simulink model "adaptive_observer_for_sin_signal_original"  (R2021b)
settings: Solver=ode4  StartTime=0.0  StopTime=simulationTime  FixedStep=0.0001  RelTol=1e-3
model workspace: external: MATLAB File D:\practice\sci\variables2n1.m (data not in the file)
values from neighbouring files (symbols this model uses):
  A = zeros(2*dimension+1 , 2*dimension+1)    [LCAD.m]
  alpha = [1,3]    [variables2n1.m]
  amp = [1;1]    [variables2n1.m]
  amp_M = [1;1]    [variables2n1.m]
  amp_M1 = 0.2    [variables2n1.m]
  bias = [0;0]    [variables2n1.m]
  bias_M = [0;0]    [variables2n1.m]
  bias_M1 = 0    [variables2n1.m]
  bigGammaZ0 = zeros(2*dimension+1, dimension)    [variables2n1.m]
  C = zeros(1, 2*dimension+1)    [LCAD.m]
  delta = C*A    [LCAD.m]    (also in stats.m = 0.05)
  dimension = 2    [variables2n1.m]
  freq = [2;3]    [variables2n1.m]
  freq_M = [1.8;3.2]    [variables2n1.m]
  freq_M1 = 20    [variables2n1.m]
  freqSwitcher = [80,150]    [variables2n1.m]
  gamma_my = 0.01    [starter3.m]
  h_my = 0.3    [starter3.m]
  initialTheta = [initialOmega(1)^2-alpha(1);     initialOmega(2)^2-alpha(2)]    [variables2n1.m]
  initialZ = [sin(phase(1)); r^2*cos(phase(1))/initialOmega(1);     sin(phase(2)); r^2*cos(phase(2))/initialOmega(2); sum(bias)]    [variables2n1.m]
  k_my = 100    [starter3.m]
  L = real((place(A',C',eigenvalues))')    [LCAD.m]
  mu = 25    [graphs.m]    (also in plot_pres4.m = 2.5; variables2n1.m = 2.5)
  noiseOrSin = 0    [variables2n1.m]
  noiseOrSwitch = 0    [variables2n1.m]
  omega1 = ones(1, length(time))*2    [graphs.m]    (also in starter3.m = 2)
  omega2 = ones(1, length(time))*3    [graphs.m]    (also in starter3.m = 3)
  omega_max = 10    [starter3.m]
  omega_min = 1    [starter3.m]
  omegaLimiter = sqrt(dimension)*maxOmega    [variables2n1.m]
  phase = [0;0]    [variables2n1.m]
  phase_M = [0;0]    [variables2n1.m]
  phase_M1 = 0    [variables2n1.m]
  r = 1.2    [variables2n1.m]
  sample_M1 = 10    [variables2n1.m]
  tau_my = 0.3    [starter3.m]
  theta0_my = [-2; 1]    [starter3.m]
  theta_real = [-c1-c2; c1*c2]    [starter3.m]
  turn_mods_on = 1    [variables2n1.m]
  zMax = 5    [variables2n1.m]
undefined symbols (not defined in the file or in its folder): G, isComplex, L1
libraries: simulink x1
(part 2 of 3)

== system adaptive_observer_for_sin_signal_original/Proposed Estimator/Subsystem ==
  Ω : Inport
  Constant1 : Constant  Value=r^2
  Divide : Product  Inputs=*/
  Gain1 : Gain  Gain=r^2
  Transpose{,1..3} (4 alike) : Math  Operator=transpose  SaturateOnIntegerOverflow=on
  Λ : Constant  Value=alpha
  Ω-Λ : Sum  Inputs=+-
  Ф : Outport
  wires:
  Divide/1 -> Ω-Λ/1
  Ω-Λ/1 -> Transpose1/1
  Ω/1 -> Divide/1
  Constant1/1 -> Divide/2
  Gain1/1 -> Transpose2/1
  Λ/1 -> Transpose/1
  Transpose/1 -> Gain1/1
  Transpose2/1 -> Ω-Λ/2
  Transpose1/1 -> Transpose3/1
  Transpose3/1 -> Ф/1

== system adaptive_observer_for_sin_signal_original/Proposed Estimator/Subsystem1 ==
  u : Inport
  Complex to Real-Imag : ComplexToRealImag
  MATLAB Function : MATLAB Function  TreatAsAtomicUnit=on
  Real-Imag to Complex : RealImagToComplex
  Switcher : Switch  Criteria=u2 ~= 0  Threshold=freqSwitcher(1)
  isComplex : Constant  Value=isComplex
  "∫Z " : Integrator  Priority=1  InitialCondition=real(initialZ)
  ∫Z 1 : Integrator  Priority=1  InitialCondition=imag(initialZ)
  Out1 : Outport
  wires:
  isComplex/1 -> Switcher/2
  u/1 -> MATLAB Function/1(zPrime), Complex to Real-Imag/1
  "∫Z "/1 -> Real-Imag to Complex/1, Switcher/1
  Switcher/1 -> Out1/1
  Complex to Real-Imag/1 -> "∫Z "/1
  Complex to Real-Imag/2 -> ∫Z 1/1
  ∫Z 1/1 -> Real-Imag to Complex/2
  Real-Imag to Complex/1 -> Switcher/3

== system adaptive_observer_for_sin_signal_original/Proposed Estimator/z' ==
  y : Inport
  Г(z) : Inport  Port=2
  Ф : Inport  Port=3
  z : Inport  Port=4
  Minus : Sum  Inputs=+-
  Product : Product  Multiplication=Matrix(*)
  S(z) : Subsystem
  Subsystem : Subsystem
  z' : Outport
  wires:
  z/1 -> Subsystem/4(z), S(z)/2(z)
  Minus/1 -> z'/1
  S(z)/1(S) -> Product/1
  Product/1 -> Minus/2
  Subsystem/1(zPreDot) -> Minus/1, Product/2, S(z)/1(zPreDot)
  Г(z)/1 -> Subsystem/1(bigGamma)
  Ф/1 -> Subsystem/2(PHI)
  y/1 -> Subsystem/3(y)

== system adaptive_observer_for_sin_signal_original/Proposed Estimator1/Frequencies estimator ==
  Ф : Inport
  ż : Inport  Port=2
  Ω in : Inport  Port=3
  z : Inport  Port=4
  y : Inport  Port=5
  Fc : Subsystem  Priority=8  TreatAsAtomicUnit=on
      settings: PortSchema="{\"entries\":[{\"content\":{\"sides\":[{\"content\":{\"connectorIds\":[\"In1\",\"In2\",\"In3\"]},\"type\":\"ConnectorPlacement.EquallySpacedRectSide\",\"uuid\":\"ef8cffdc-1e6f-42c0-8cb3-bf318ca182f8\"},{\"content\":{\"connectorIds\":[\"Out1\"],\"side\":\"RIGHT\"},\"type\":\"ConnectorPlacement.EquallySpacedRectSide\",\"uuid\":\"a9c7e5b7-281a-47aa-808a-eb2877f3eee0\"},{\"content\":{\"connectorIds\":[\"In4\"],\"side\":\"TOP\"},\"type\":\"ConnectorPlacement.EquallySpacedRectSide\",\"uuid\":\"7bb4f6b5-7deb-4e08-9b2d-b96cfbb2c85e\"},{\"content\":{\"connectorIds\":[],\"side\":\"BOTTOM\"},\"type\":\"ConnectorPlacement.EquallySpacedRectSide\",\"uuid\":\"d628d464-6f95-4c60-8de5-a9188665a8a2\"}]},\"type\":\"ConnectorPlacement.EquallySpacedConnector\",\"uuid\":\"64fccc24-315d-40ff-920f-bd434d551c1a\"}],\"packageUris\":[\"http://schema.mathworks.com/mf0/Connector/R2020b\"],\"version\":\"1.0\"}"
  Fu : Subsystem  Priority=9  TreatAsAtomicUnit=on
      settings: PortSchema="{\"entries\":[{\"content\":{\"sides\":[{\"content\":{\"connectorIds\":[\"In1\",\"In2\"]},\"type\":\"ConnectorPlacement.EquallySpacedRectSide\",\"uuid\":\"56415c13-d553-4f88-94d3-75bcdc800e4b\"},{\"content\":{\"connectorIds\":[\"Out1\"],\"side\":\"RIGHT\"},\"type\":\"ConnectorPlacement.EquallySpacedRectSide\",\"uuid\":\"a1bdd2d2-4e49-40cb-b0b7-1df5316e4510\"},{\"content\":{\"connectorIds\":[\"In3\"],\"side\":\"TOP\"},\"type\":\"ConnectorPlacement.EquallySpacedRectSide\",\"uuid\":\"59b6ba3d-4a55-43e8-9b14-0d873cc3c9ca\"},{\"content\":{\"connectorIds\":[\"In4\",\"In5\"],\"side\":\"BOTTOM\"},\"type\":\"ConnectorPlacement.EquallySpacedRectSide\",\"uuid\":\"cb3db39e-f643-4fe7-a27f-76e86359c78d\"}]},\"type\":\"ConnectorPlacement.EquallySpacedConnector\",\"uuid\":\"fdf2e112-ecff-41aa-a5cb-d527a9dd51a8\"}],\"packageUris\":[\"http://schema.mathworks.com/mf0/Connector/R2020b\"],\"version\":\"1.0\"}"
  Ω : Subsystem  Priority=5  TreatAsAtomicUnit=on
      settings: PortSchema="{\"entries\":[{\"content\":{\"sides\":[{\"content\":{\"connectorIds\":[\"In1\",\"In2\"]},\"type\":\"ConnectorPlacement.EquallySpacedRectSide\",\"uuid\":\"0172ca52-64e8-432c-895c-e5829558e278\"},{\"content\":{\"connectorIds\":[\"Out1\"],\"side\":\"RIGHT\"},\"type\":\"ConnectorPlacement.EquallySpacedRectSide\",\"uuid\":\"c83f4e01-5d94-498a-a9de-b4a302d500ab\"},{\"content\":{\"connectorIds\":[\"In3\"],\"side\":\"TOP\"},\"type\":\"ConnectorPlacement.EquallySpacedRectSide\",\"uuid\":\"3a6496e3-470c-4361-9f8f-cd28e1556398\"}]},\"type\":\"ConnectorPlacement.EquallySpacedConnector\",\"uuid\":\"b738ec8a-20ee-4a0a-8362-4988f331d970\"}],\"packageUris\":[\"http://schema.mathworks.com/mf0/Connector/R2020b\"],\"version\":\"1.0\"}"
  θ' : Subsystem  Priority=10  TreatAsAtomicUnit=on
      settings: PortSchema="{\"entries\":[{\"content\":{\"sides\":[{\"content\":{\"connectorIds\":[\"In1\"]},\"type\":\"ConnectorPlacement.EquallySpacedRectSide\",\"uuid\":\"9184f415-d771-478b-8114-38f854f6aad6\"},{\"content\":{\"connectorIds\":[\"Out1\"],\"side\":\"RIGHT\"},\"type\":\"ConnectorPlacement.EquallySpacedRectSide\",\"uuid\":\"399c2935-e635-4d1c-9ba7-451eea57bae3\"},{\"content\":{\"connectorIds\":[\"In2\"],\"side\":\"TOP\"},\"type\":\"ConnectorPlacement.EquallySpacedRectSide\",\"uuid\":\"bdc6ec05-8dca-4996-ba70-702aa29fd179\"}]},\"type\":\"ConnectorPlacement.EquallySpacedConnector\",\"uuid\":\"fa68c3f3-8285-4ee8-b99d-908dba81143c\"}],\"packageUris\":[\"http://schema.mathworks.com/mf0/Connector/R2020b\"],\"version\":\"1.0\"}"
  г(z) : Selector  InputPortWidth=2*dimension+1  IndexOptions=Index vector (dialog)  Indices=2:2:2*dimension  OutputSizes=1
  "∫θ " : Integrator  Priority=3  InitialCondition=initialTheta
  Ω out : Outport
  wires:
  Ф/1 -> Fu/1(Ф), Fc/3(Ф)
  y/1 -> Ω/2(y), Fu/5(y)
  z/1 -> г(z)/1, Fu/2(z), Fc/1(z)
  г(z)/1 -> Fc/4(Г(z)), Ω/3(г(z)), Fu/4(г(z))
  Ω in/1 -> Fc/2(Ω)
  ż/1 -> Fu/3(ż)
  "∫θ "/1 -> Ω/1(θ)
  Ω/1(Ω) -> Ω out/1
  Fc/1(Fc) -> θ'/2(Fc)
  Fu/1(Fu) -> θ'/1(Fu)
  θ'/1(θ') -> "∫θ "/1

== system adaptive_observer_for_sin_signal_original/Proposed Estimator1/Subsystem ==
  Ω : Inport
  Constant1 : Constant  Value=r^2
  Divide : Product  Inputs=*/
  Gain1 : Gain  Gain=r^2
  Transpose{,1..3} (4 alike) : Math  Operator=transpose  SaturateOnIntegerOverflow=on
  Λ : Constant  Value=alpha
  Ω-Λ : Sum  Inputs=+-
  Ф : Outport
  wires:
  Divide/1 -> Ω-Λ/1
  Ω-Λ/1 -> Transpose1/1
  Ω/1 -> Divide/1
  Constant1/1 -> Divide/2
  Gain1/1 -> Transpose2/1
  Λ/1 -> Transpose/1
  Transpose/1 -> Gain1/1
  Transpose2/1 -> Ω-Λ/2
  Transpose1/1 -> Transpose3/1
  Transpose3/1 -> Ф/1

== system adaptive_observer_for_sin_signal_original/Proposed Estimator1/Subsystem1 ==
  u : Inport
  Complex to Real-Imag : ComplexToRealImag
  MATLAB Function : MATLAB Function  TreatAsAtomicUnit=on
  Real-Imag to Complex : RealImagToComplex
  Switcher : Switch  Criteria=u2 ~= 0  Threshold=freqSwitcher(1)
  isComplex : Constant  Value=isComplex
  "∫Z " : Integrator  Priority=1  InitialCondition=real(initialZ)
  ∫Z 1 : Integrator  Priority=1  InitialCondition=imag(initialZ)
  Out1 : Outport
  wires:
  isComplex/1 -> Switcher/2
  u/1 -> MATLAB Function/1(zPrime), Complex to Real-Imag/1
  "∫Z "/1 -> Real-Imag to Complex/1, Switcher/1
  Switcher/1 -> Out1/1
  Complex to Real-Imag/1 -> "∫Z "/1
  Complex to Real-Imag/2 -> ∫Z 1/1
  ∫Z 1/1 -> Real-Imag to Complex/2
  Real-Imag to Complex/1 -> Switcher/3

== system adaptive_observer_for_sin_signal_original/Proposed Estimator1/z' ==
  y : Inport
  Г(z) : Inport  Port=2
  Ф : Inport  Port=3
  z : Inport  Port=4
  Minus : Sum  Inputs=+-
  Product : Product  Multiplication=Matrix(*)
  S(z) : Subsystem
  Subsystem : Subsystem
  z' : Outport
  wires:
  z/1 -> Subsystem/4(z), S(z)/2(z)
  Minus/1 -> z'/1
  S(z)/1(S) -> Product/1
  Product/1 -> Minus/2
  Subsystem/1(zPreDot) -> Minus/1, Product/2, S(z)/1(zPreDot)
  Г(z)/1 -> Subsystem/1(bigGamma)
  Ф/1 -> Subsystem/2(PHI)
  y/1 -> Subsystem/3(y)

== system adaptive_observer_for_sin_signal_original/Estimator mu=10/Frequencies estimator/Fc ==
  note: Определение максимального S
  note: Переключатель ограничителя Fc
  z : Inport
  Ω : Inport  Port=2
  Ф : Inport  Port=3
  Г(z) : Inport  Port=4
  Clock : Clock
  Constant : Constant  Value=mu(4)
  Scope2 : Scope
  Unary Minus : UnaryMinus
  max S1 : MATLAB Function  TreatAsAtomicUnit=on
  product : Product  Inputs=3
  ||Ω|| : MATLAB Function  TreatAsAtomicUnit=on
  "||Ω|| >= Ω cap ? " : RelationalOperator  OutDataTypeStr=boolean  RndMeth=Simplest
  Ψ : MATLAB Function  TreatAsAtomicUnit=on
  Ω * √n : Constant  Value=omegaLimiter
  Ω / Ω cap : Product  Inputs=*/
  Fc : Outport
  wires:
  Ф/1 -> max S1/3(PHI)
  Ω/1 -> max S1/1(bigOmega), Ω / Ω cap/1, ||Ω||/1(bigOmega)
  max S1/1(maxS) -> product/3, Scope2/1
  Г(z)/1 -> max S1/4(gammaZ)
  z/1 -> max S1/2(z)
  ||Ω||/1(normOmega) -> "||Ω|| >= Ω cap ? "/1
  Ω * √n/1 -> Ω / Ω cap/2, "||Ω|| >= Ω cap ? "/2
  "||Ω|| >= Ω cap ? "/1 -> Ψ/1(isGreater)
  Ψ/1(Psi) -> product/1
  Ω / Ω cap/1 -> product/2
  product/1 -> Unary Minus/1
  Unary Minus/1 -> Fc/1
  Clock/1 -> max S1/5(t)
  Constant/1 -> max S1/6(mu)

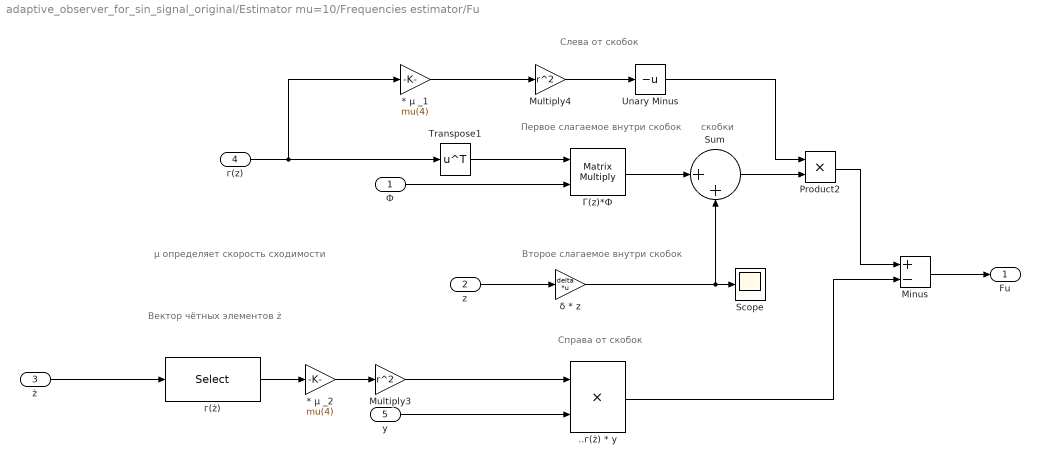
== system adaptive_observer_for_sin_signal_original/Estimator mu=10/Frequencies estimator/Fu ==
  note: Вектор чётных элементов ż
  note: μ определяет скорость сходимости
  note: скобки
  note: Первое слагаемое внутри скобок
  note: Второе слагаемое внутри скобок
  note: Слева от скобок
  note: Справа от скобок
  Ф : Inport
  z : Inport  Port=2
  ż : Inport  Port=3
  г(z) : Inport  Port=4
  y : Inport  Port=5
  * μ _1 : Gain  Gain=mu(4)
  * μ _2 : Gain  Gain=mu(4)
  ..г(ż) * y : Product
  Minus : Sum  Inputs=+-
  Multiply3 : Gain  Gain=r^2
  Multiply4 : Gain  Gain=r^2
  Product2 : Product
  Scope : Scope
  Sum : Sum  Inputs=|++
  Transpose1 : Math  Operator=transpose  SaturateOnIntegerOverflow=on
  Unary Minus : UnaryMinus
  δ * z : Gain  Gain=delta  Multiplication=Matrix(K*u)
  Г(z)*Ф : Product  Multiplication=Matrix(*)
  г(ż) : Selector  InputPortWidth=2*dimension+1  IndexOptions=Index vector (dialog)  Indices=2:2:2*dimension  OutputSizes=1
  Fu : Outport
  wires:
  ż/1 -> г(ż)/1
  г(z)/1 -> * μ _1/1, Transpose1/1
  * μ _2/1 -> Multiply3/1
  г(ż)/1 -> * μ _2/1
  Multiply3/1 -> ..г(ż) * y/1
  y/1 -> ..г(ż) * y/2
  Transpose1/1 -> Г(z)*Ф/1
  * μ _1/1 -> Multiply4/1
  Multiply4/1 -> Unary Minus/1
  z/1 -> δ * z/1
  Г(z)*Ф/1 -> Sum/1
  δ * z/1 -> Scope/1, Sum/2
  Unary Minus/1 -> Product2/1
  Sum/1 -> Product2/2
  Product2/1 -> Minus/1
  ..г(ż) * y/1 -> Minus/2
  Minus/1 -> Fu/1
  Ф/1 -> Г(z)*Ф/2

== system adaptive_observer_for_sin_signal_original/Estimator mu=10/Frequencies estimator/Ω ==
  note: Оценка частот в момент времени t
  θ : Inport
  y : Inport  Port=2
  г(z) : Inport  Port=3
  ..г(z)*y : Product
  Gain : Gain  Gain=r^2
  Sum : Sum  Inputs=|++
  μ : Gain  Gain=mu(4)
  Ω : Outport
  wires:
  г(z)/1 -> Gain/1
  Gain/1 -> μ/1
  μ/1 -> ..г(z)*y/1
  y/1 -> ..г(z)*y/2
  ..г(z)*y/1 -> Sum/1
  θ/1 -> Sum/2
  Sum/1 -> Ω/1

== system adaptive_observer_for_sin_signal_original/Estimator mu=10/Frequencies estimator/θ' ==
  note: Образует основу θ'
  note: Удерживает Ω в области определения
  Fu : Inport
  Fc : Inport  Port=2
  Sum : Sum  Inputs=|++
  θ' : Outport
  wires:
  Fu/1 -> Sum/2
  Sum/1 -> θ'/1
  Fc/1 -> Sum/1

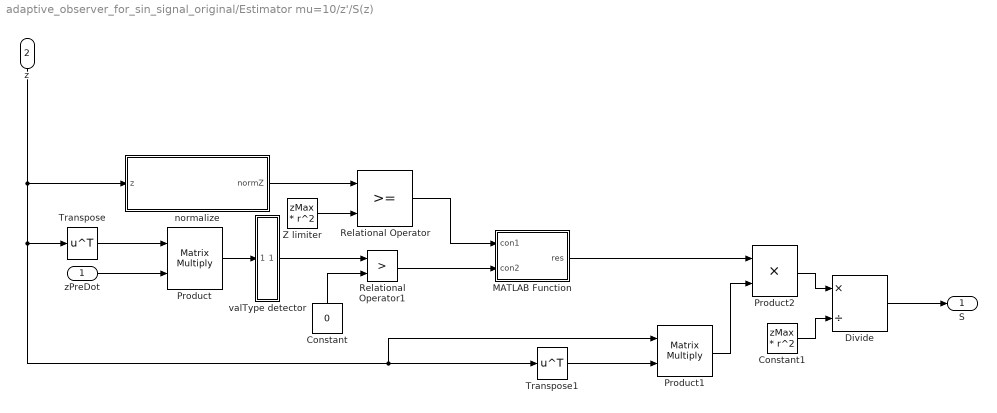
== system adaptive_observer_for_sin_signal_original/Estimator mu=10/z'/S(z) ==
  zPreDot : Inport
  z : Inport  Port=2
  Constant : Constant  Value=0
  Constant1 : Constant  Value=zMax * r^2
  Divide : Product  Inputs=*/
  MATLAB Function : MATLAB Function  TreatAsAtomicUnit=on
  Product : Product  Multiplication=Matrix(*)
  Product1 : Product  Multiplication=Matrix(*)
  Product2 : Product
  Relational Operator : RelationalOperator  OutDataTypeStr=boolean  RndMeth=Simplest
  Relational Operator1 : RelationalOperator  Operator=>  OutDataTypeStr=boolean  RndMeth=Simplest
  Transpose : Math  Operator=transpose  SaturateOnIntegerOverflow=on
  Transpose1 : Math  Operator=transpose  SaturateOnIntegerOverflow=on
  Z limiter : Constant  Value=zMax * r^2
  normalize : MATLAB Function  TreatAsAtomicUnit=on
  valType detector : MATLAB Function  TreatAsAtomicUnit=on
  S : Outport
  wires:
  Z limiter/1 -> Relational Operator/2
  normalize/1(normZ) -> Relational Operator/1
  Relational Operator/1 -> MATLAB Function/1(con1)
  z/1 -> Product1/1, Transpose1/1, Transpose/1, normalize/1(z)
  Transpose/1 -> Product/1
  zPreDot/1 -> Product/2
  Product/1 -> valType detector/1(multiplied)
  Constant/1 -> Relational Operator1/2
  Relational Operator1/1 -> MATLAB Function/2(con2)
  MATLAB Function/1(res) -> Product2/1
  Transpose1/1 -> Product1/2
  Product1/1 -> Product2/2
  Product2/1 -> Divide/1
  Constant1/1 -> Divide/2
  Divide/1 -> S/1
  valType detector/1(filtered) -> Relational Operator1/1

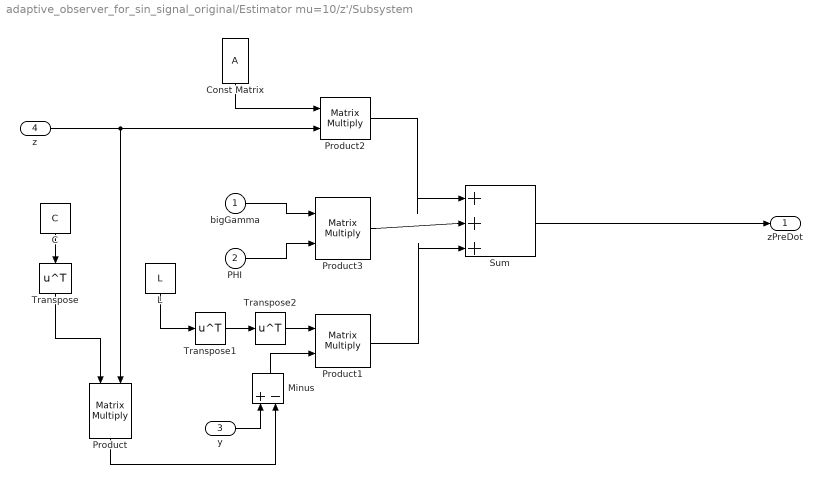
== system adaptive_observer_for_sin_signal_original/Estimator mu=10/z'/Subsystem ==
  bigGamma : Inport
  PHI : Inport  Port=2
  y : Inport  Port=3
  z : Inport  Port=4
  C : Constant  Value=C
  Const Matrix : Constant  Value=A
  L : Constant  Value=L
  Minus : Sum  Inputs=+-
  Product{,1..3} (4 alike) : Product  Multiplication=Matrix(*)
  Sum : Sum  Inputs=|+++
  Transpose : Math  Operator=transpose  SaturateOnIntegerOverflow=on
  Transpose1 : Math  Operator=transpose  SaturateOnIntegerOverflow=on
  Transpose2 : Math  Operator=transpose  SaturateOnIntegerOverflow=on
  zPreDot : Outport
  wires:
  z/1 -> Product2/2, Product/2
  Sum/1 -> zPreDot/1
  C/1 -> Transpose/1
  y/1 -> Minus/1
  Product/1 -> Minus/2
  L/1 -> Transpose1/1
  Minus/1 -> Product1/2
  Const Matrix/1 -> Product2/1
  bigGamma/1 -> Product3/1
  PHI/1 -> Product3/2
  Product2/1 -> Sum/1
  Product3/1 -> Sum/2
  Product1/1 -> Sum/3
  Transpose/1 -> Product/1
  Transpose2/1 -> Product1/1
  Transpose1/1 -> Transpose2/1

== system adaptive_observer_for_sin_signal_original/Estimator mu=2.5/Frequencies estimator/Fc ==
  note: Определение максимального S
  note: Переключатель ограничителя Fc
  z : Inport
  Ω : Inport  Port=2
  Ф : Inport  Port=3
  Г(z) : Inport  Port=4
  Clock : Clock
  Constant : Constant  Value=mu(2)
  Scope2 : Scope
  Unary Minus : UnaryMinus
  max S1 : MATLAB Function  TreatAsAtomicUnit=on
  product : Product  Inputs=3
  ||Ω|| : MATLAB Function  TreatAsAtomicUnit=on
  "||Ω|| >= Ω cap ? " : RelationalOperator  OutDataTypeStr=boolean  RndMeth=Simplest
  Ψ : MATLAB Function  TreatAsAtomicUnit=on
  Ω * √n : Constant  Value=omegaLimiter
  Ω / Ω cap : Product  Inputs=*/
  Fc : Outport
  wires:
  Ф/1 -> max S1/3(PHI)
  Ω/1 -> max S1/1(bigOmega), Ω / Ω cap/1, ||Ω||/1(bigOmega)
  max S1/1(maxS) -> product/3, Scope2/1
  Г(z)/1 -> max S1/4(gammaZ)
  z/1 -> max S1/2(z)
  ||Ω||/1(normOmega) -> "||Ω|| >= Ω cap ? "/1
  Ω * √n/1 -> Ω / Ω cap/2, "||Ω|| >= Ω cap ? "/2
  "||Ω|| >= Ω cap ? "/1 -> Ψ/1(isGreater)
  Ψ/1(Psi) -> product/1
  Ω / Ω cap/1 -> product/2
  product/1 -> Unary Minus/1
  Unary Minus/1 -> Fc/1
  Clock/1 -> max S1/5(t)
  Constant/1 -> max S1/6(mu)

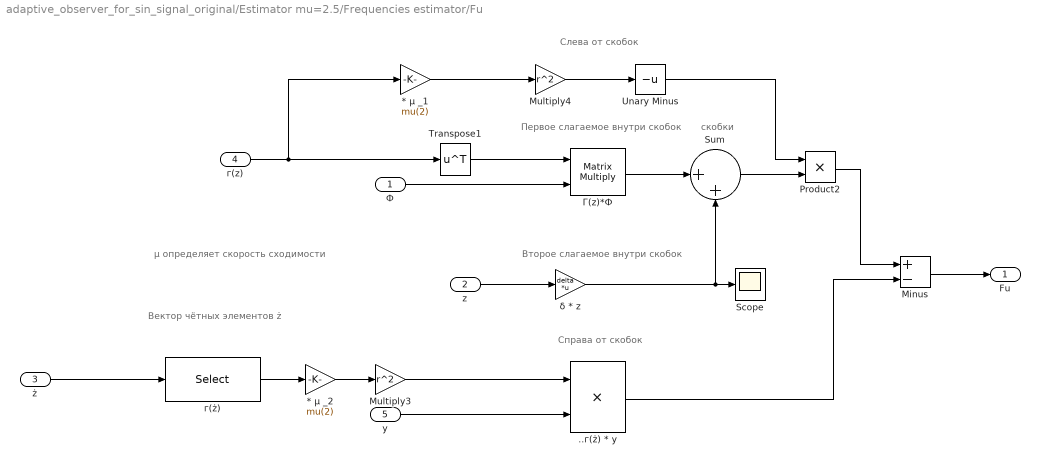
== system adaptive_observer_for_sin_signal_original/Estimator mu=2.5/Frequencies estimator/Fu ==
  note: Вектор чётных элементов ż
  note: μ определяет скорость сходимости
  note: скобки
  note: Первое слагаемое внутри скобок
  note: Второе слагаемое внутри скобок
  note: Слева от скобок
  note: Справа от скобок
  Ф : Inport
  z : Inport  Port=2
  ż : Inport  Port=3
  г(z) : Inport  Port=4
  y : Inport  Port=5
  * μ _1 : Gain  Gain=mu(2)
  * μ _2 : Gain  Gain=mu(2)
  ..г(ż) * y : Product
  Minus : Sum  Inputs=+-
  Multiply3 : Gain  Gain=r^2
  Multiply4 : Gain  Gain=r^2
  Product2 : Product
  Scope : Scope
  Sum : Sum  Inputs=|++
  Transpose1 : Math  Operator=transpose  SaturateOnIntegerOverflow=on
  Unary Minus : UnaryMinus
  δ * z : Gain  Gain=delta  Multiplication=Matrix(K*u)
  Г(z)*Ф : Product  Multiplication=Matrix(*)
  г(ż) : Selector  InputPortWidth=2*dimension+1  IndexOptions=Index vector (dialog)  Indices=2:2:2*dimension  OutputSizes=1
  Fu : Outport
  wires:
  ż/1 -> г(ż)/1
  г(z)/1 -> * μ _1/1, Transpose1/1
  * μ _2/1 -> Multiply3/1
  г(ż)/1 -> * μ _2/1
  Multiply3/1 -> ..г(ż) * y/1
  y/1 -> ..г(ż) * y/2
  Transpose1/1 -> Г(z)*Ф/1
  * μ _1/1 -> Multiply4/1
  Multiply4/1 -> Unary Minus/1
  z/1 -> δ * z/1
  Г(z)*Ф/1 -> Sum/1
  δ * z/1 -> Scope/1, Sum/2
  Unary Minus/1 -> Product2/1
  Sum/1 -> Product2/2
  Product2/1 -> Minus/1
  ..г(ż) * y/1 -> Minus/2
  Minus/1 -> Fu/1
  Ф/1 -> Г(z)*Ф/2

== system adaptive_observer_for_sin_signal_original/Estimator mu=2.5/Frequencies estimator/Ω ==
  note: Оценка частот в момент времени t
  θ : Inport
  y : Inport  Port=2
  г(z) : Inport  Port=3
  ..г(z)*y : Product
  Gain : Gain  Gain=r^2
  Sum : Sum  Inputs=|++
  μ : Gain  Gain=mu(2)
  Ω : Outport
  wires:
  г(z)/1 -> Gain/1
  Gain/1 -> μ/1
  μ/1 -> ..г(z)*y/1
  y/1 -> ..г(z)*y/2
  ..г(z)*y/1 -> Sum/1
  θ/1 -> Sum/2
  Sum/1 -> Ω/1

== system adaptive_observer_for_sin_signal_original/Estimator mu=2.5/Frequencies estimator/θ' ==
  note: Образует основу θ'
  note: Удерживает Ω в области определения
  Fu : Inport
  Fc : Inport  Port=2
  Sum : Sum  Inputs=|++
  θ' : Outport
  wires:
  Fu/1 -> Sum/2
  Sum/1 -> θ'/1
  Fc/1 -> Sum/1

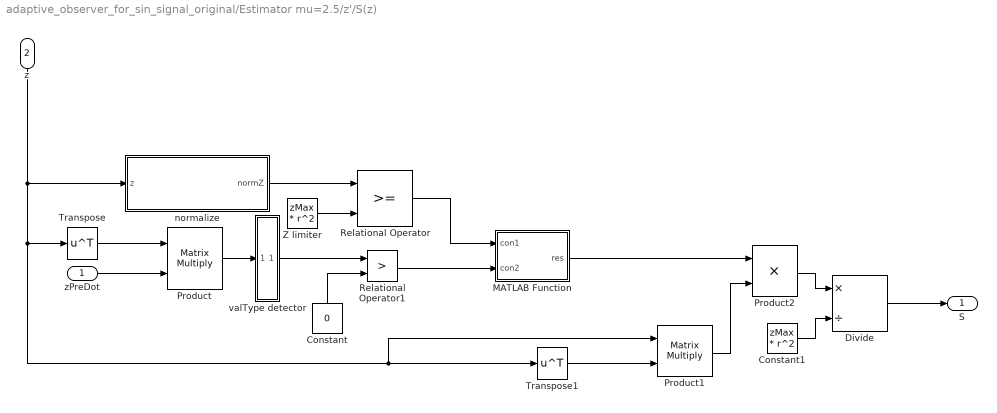
== system adaptive_observer_for_sin_signal_original/Estimator mu=2.5/z'/S(z) ==
  zPreDot : Inport
  z : Inport  Port=2
  Constant : Constant  Value=0
  Constant1 : Constant  Value=zMax * r^2
  Divide : Product  Inputs=*/
  MATLAB Function : MATLAB Function  TreatAsAtomicUnit=on
  Product : Product  Multiplication=Matrix(*)
  Product1 : Product  Multiplication=Matrix(*)
  Product2 : Product
  Relational Operator : RelationalOperator  OutDataTypeStr=boolean  RndMeth=Simplest
  Relational Operator1 : RelationalOperator  Operator=>  OutDataTypeStr=boolean  RndMeth=Simplest
  Transpose : Math  Operator=transpose  SaturateOnIntegerOverflow=on
  Transpose1 : Math  Operator=transpose  SaturateOnIntegerOverflow=on
  Z limiter : Constant  Value=zMax * r^2
  normalize : MATLAB Function  TreatAsAtomicUnit=on
  valType detector : MATLAB Function  TreatAsAtomicUnit=on
  S : Outport
  wires:
  Z limiter/1 -> Relational Operator/2
  normalize/1(normZ) -> Relational Operator/1
  Relational Operator/1 -> MATLAB Function/1(con1)
  z/1 -> Product1/1, Transpose1/1, Transpose/1, normalize/1(z)
  Transpose/1 -> Product/1
  zPreDot/1 -> Product/2
  Product/1 -> valType detector/1(multiplied)
  Constant/1 -> Relational Operator1/2
  Relational Operator1/1 -> MATLAB Function/2(con2)
  MATLAB Function/1(res) -> Product2/1
  Transpose1/1 -> Product1/2
  Product1/1 -> Product2/2
  Product2/1 -> Divide/1
  Constant1/1 -> Divide/2
  Divide/1 -> S/1
  valType detector/1(filtered) -> Relational Operator1/1

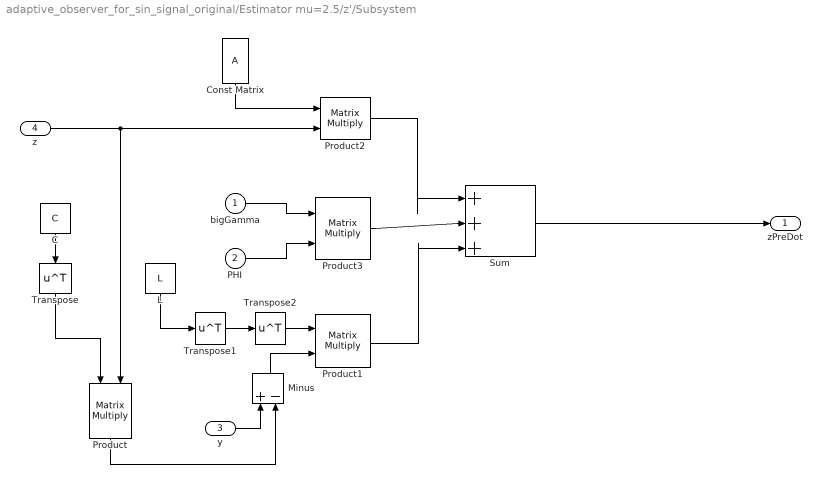
== system adaptive_observer_for_sin_signal_original/Estimator mu=2.5/z'/Subsystem ==
  bigGamma : Inport
  PHI : Inport  Port=2
  y : Inport  Port=3
  z : Inport  Port=4
  C : Constant  Value=C
  Const Matrix : Constant  Value=A
  L : Constant  Value=L
  Minus : Sum  Inputs=+-
  Product{,1..3} (4 alike) : Product  Multiplication=Matrix(*)
  Sum : Sum  Inputs=|+++
  Transpose : Math  Operator=transpose  SaturateOnIntegerOverflow=on
  Transpose1 : Math  Operator=transpose  SaturateOnIntegerOverflow=on
  Transpose2 : Math  Operator=transpose  SaturateOnIntegerOverflow=on
  zPreDot : Outport
  wires:
  z/1 -> Product2/2, Product/2
  Sum/1 -> zPreDot/1
  C/1 -> Transpose/1
  y/1 -> Minus/1
  Product/1 -> Minus/2
  L/1 -> Transpose1/1
  Minus/1 -> Product1/2
  Const Matrix/1 -> Product2/1
  bigGamma/1 -> Product3/1
  PHI/1 -> Product3/2
  Product2/1 -> Sum/1
  Product3/1 -> Sum/2
  Product1/1 -> Sum/3
  Transpose/1 -> Product/1
  Transpose2/1 -> Product1/1
  Transpose1/1 -> Transpose2/1

== system adaptive_observer_for_sin_signal_original/Estimator mu=5/Frequencies estimator/Fc ==
  note: Определение максимального S
  note: Переключатель ограничителя Fc
  z : Inport
  Ω : Inport  Port=2
  Ф : Inport  Port=3
  Г(z) : Inport  Port=4
  Clock : Clock
  Constant : Constant  Value=mu(3)
  Scope2 : Scope
  Unary Minus : UnaryMinus
  max S1 : MATLAB Function  TreatAsAtomicUnit=on
  product : Product  Inputs=3
  ||Ω|| : MATLAB Function  TreatAsAtomicUnit=on
  "||Ω|| >= Ω cap ? " : RelationalOperator  OutDataTypeStr=boolean  RndMeth=Simplest
  Ψ : MATLAB Function  TreatAsAtomicUnit=on
  Ω * √n : Constant  Value=omegaLimiter
  Ω / Ω cap : Product  Inputs=*/
  Fc : Outport
  wires:
  Ф/1 -> max S1/3(PHI)
  Ω/1 -> max S1/1(bigOmega), Ω / Ω cap/1, ||Ω||/1(bigOmega)
  max S1/1(maxS) -> product/3, Scope2/1
  Г(z)/1 -> max S1/4(gammaZ)
  z/1 -> max S1/2(z)
  ||Ω||/1(normOmega) -> "||Ω|| >= Ω cap ? "/1
  Ω * √n/1 -> Ω / Ω cap/2, "||Ω|| >= Ω cap ? "/2
  "||Ω|| >= Ω cap ? "/1 -> Ψ/1(isGreater)
  Ψ/1(Psi) -> product/1
  Ω / Ω cap/1 -> product/2
  product/1 -> Unary Minus/1
  Unary Minus/1 -> Fc/1
  Clock/1 -> max S1/5(t)
  Constant/1 -> max S1/6(mu)

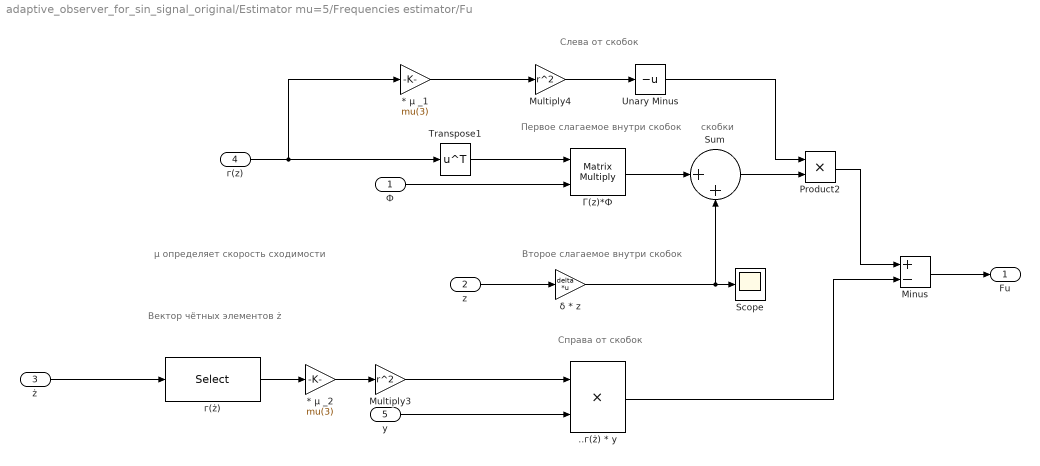
== system adaptive_observer_for_sin_signal_original/Estimator mu=5/Frequencies estimator/Fu ==
  note: Вектор чётных элементов ż
  note: μ определяет скорость сходимости
  note: скобки
  note: Первое слагаемое внутри скобок
  note: Второе слагаемое внутри скобок
  note: Слева от скобок
  note: Справа от скобок
  Ф : Inport
  z : Inport  Port=2
  ż : Inport  Port=3
  г(z) : Inport  Port=4
  y : Inport  Port=5
  * μ _1 : Gain  Gain=mu(3)
  * μ _2 : Gain  Gain=mu(3)
  ..г(ż) * y : Product
  Minus : Sum  Inputs=+-
  Multiply3 : Gain  Gain=r^2
  Multiply4 : Gain  Gain=r^2
  Product2 : Product
  Scope : Scope
  Sum : Sum  Inputs=|++
  Transpose1 : Math  Operator=transpose  SaturateOnIntegerOverflow=on
  Unary Minus : UnaryMinus
  δ * z : Gain  Gain=delta  Multiplication=Matrix(K*u)
  Г(z)*Ф : Product  Multiplication=Matrix(*)
  г(ż) : Selector  InputPortWidth=2*dimension+1  IndexOptions=Index vector (dialog)  Indices=2:2:2*dimension  OutputSizes=1
  Fu : Outport
  wires:
  ż/1 -> г(ż)/1
  г(z)/1 -> * μ _1/1, Transpose1/1
  * μ _2/1 -> Multiply3/1
  г(ż)/1 -> * μ _2/1
  Multiply3/1 -> ..г(ż) * y/1
  y/1 -> ..г(ż) * y/2
  Transpose1/1 -> Г(z)*Ф/1
  * μ _1/1 -> Multiply4/1
  Multiply4/1 -> Unary Minus/1
  z/1 -> δ * z/1
  Г(z)*Ф/1 -> Sum/1
  δ * z/1 -> Scope/1, Sum/2
  Unary Minus/1 -> Product2/1
  Sum/1 -> Product2/2
  Product2/1 -> Minus/1
  ..г(ż) * y/1 -> Minus/2
  Minus/1 -> Fu/1
  Ф/1 -> Г(z)*Ф/2

== system adaptive_observer_for_sin_signal_original/Estimator mu=5/Frequencies estimator/Ω ==
  note: Оценка частот в момент времени t
  θ : Inport
  y : Inport  Port=2
  г(z) : Inport  Port=3
  ..г(z)*y : Product
  Gain : Gain  Gain=r^2
  Sum : Sum  Inputs=|++
  μ : Gain  Gain=mu(3)
  Ω : Outport
  wires:
  г(z)/1 -> Gain/1
  Gain/1 -> μ/1
  μ/1 -> ..г(z)*y/1
  y/1 -> ..г(z)*y/2
  ..г(z)*y/1 -> Sum/1
  θ/1 -> Sum/2
  Sum/1 -> Ω/1

== system adaptive_observer_for_sin_signal_original/Estimator mu=5/Frequencies estimator/θ' ==
  note: Образует основу θ'
  note: Удерживает Ω в области определения
  Fu : Inport
  Fc : Inport  Port=2
  Sum : Sum  Inputs=|++
  θ' : Outport
  wires:
  Fu/1 -> Sum/2
  Sum/1 -> θ'/1
  Fc/1 -> Sum/1

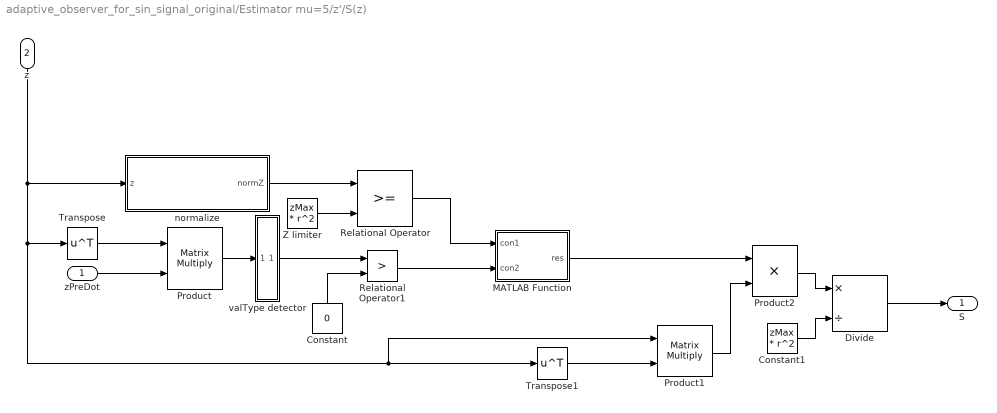
== system adaptive_observer_for_sin_signal_original/Estimator mu=5/z'/S(z) ==
  zPreDot : Inport
  z : Inport  Port=2
  Constant : Constant  Value=0
  Constant1 : Constant  Value=zMax * r^2
  Divide : Product  Inputs=*/
  MATLAB Function : MATLAB Function  TreatAsAtomicUnit=on
  Product : Product  Multiplication=Matrix(*)
  Product1 : Product  Multiplication=Matrix(*)
  Product2 : Product
  Relational Operator : RelationalOperator  OutDataTypeStr=boolean  RndMeth=Simplest
  Relational Operator1 : RelationalOperator  Operator=>  OutDataTypeStr=boolean  RndMeth=Simplest
  Transpose : Math  Operator=transpose  SaturateOnIntegerOverflow=on
  Transpose1 : Math  Operator=transpose  SaturateOnIntegerOverflow=on
  Z limiter : Constant  Value=zMax * r^2
  normalize : MATLAB Function  TreatAsAtomicUnit=on
  valType detector : MATLAB Function  TreatAsAtomicUnit=on
  S : Outport
  wires:
  Z limiter/1 -> Relational Operator/2
  normalize/1(normZ) -> Relational Operator/1
  Relational Operator/1 -> MATLAB Function/1(con1)
  z/1 -> Product1/1, Transpose1/1, Transpose/1, normalize/1(z)
  Transpose/1 -> Product/1
  zPreDot/1 -> Product/2
  Product/1 -> valType detector/1(multiplied)
  Constant/1 -> Relational Operator1/2
  Relational Operator1/1 -> MATLAB Function/2(con2)
  MATLAB Function/1(res) -> Product2/1
  Transpose1/1 -> Product1/2
  Product1/1 -> Product2/2
  Product2/1 -> Divide/1
  Constant1/1 -> Divide/2
  Divide/1 -> S/1
  valType detector/1(filtered) -> Relational Operator1/1

== system adaptive_observer_for_sin_signal_original/Estimator mu=5/z'/Subsystem ==
  bigGamma : Inport
  PHI : Inport  Port=2
  y : Inport  Port=3
  z : Inport  Port=4
  C : Constant  Value=C
  Const Matrix : Constant  Value=A
  L : Constant  Value=L
  Minus : Sum  Inputs=+-
  Product{,1..3} (4 alike) : Product  Multiplication=Matrix(*)
  Sum : Sum  Inputs=|+++
  Transpose : Math  Operator=transpose  SaturateOnIntegerOverflow=on
  Transpose1 : Math  Operator=transpose  SaturateOnIntegerOverflow=on
  Transpose2 : Math  Operator=transpose  SaturateOnIntegerOverflow=on
  zPreDot : Outport
  wires:
  z/1 -> Product2/2, Product/2
  Sum/1 -> zPreDot/1
  C/1 -> Transpose/1
  y/1 -> Minus/1
  Product/1 -> Minus/2
  L/1 -> Transpose1/1
  Minus/1 -> Product1/2
  Const Matrix/1 -> Product2/1
  bigGamma/1 -> Product3/1
  PHI/1 -> Product3/2
  Product2/1 -> Sum/1
  Product3/1 -> Sum/2
  Product1/1 -> Sum/3
  Transpose/1 -> Product/1
  Transpose2/1 -> Product1/1
  Transpose1/1 -> Transpose2/1

== system adaptive_observer_for_sin_signal_original/FT Ved/Gradient1/W ==
  PHI : Inport
  Gain1 : Gain  Gain=-gamma_my
  Integrator2 : Integrator  InitialCondition=1
  Product2 : Product  Inputs=3
  W : Outport  VectorParamsAs1DForOutWhenUnconnected=off
  wires:
  PHI/1 -> Product2/2, Product2/1
  Integrator2/1 -> Product2/3, W/1
  Product2/1 -> Gain1/1
  Gain1/1 -> Integrator2/1

== system adaptive_observer_for_sin_signal_original/Proposed Estimator/Frequencies estimator/Fc ==
  note: Определение максимального S
  note: Переключатель ограничителя Fc
  z : Inport
  Ω : Inport  Port=2
  Ф : Inport  Port=3
  Г(z) : Inport  Port=4
  Clock : Clock
  Scope2 : Scope
  Unary Minus : UnaryMinus
  max S : MATLAB Function  TreatAsAtomicUnit=on
  mu : Constant  Value=mu
  product : Product  Inputs=3
  ||Ω|| : MATLAB Function  TreatAsAtomicUnit=on
  "||Ω|| >= Ω cap ? " : RelationalOperator  OutDataTypeStr=boolean  RndMeth=Simplest
  Ψ : MATLAB Function  TreatAsAtomicUnit=on
  Ω * √n : Constant  Value=omegaLimiter
  Ω / Ω cap : Product  Inputs=*/
  Fc : Outport
  wires:
  Ф/1 -> max S/3(PHI)
  Ω/1 -> max S/1(bigOmega), Ω / Ω cap/1, ||Ω||/1(bigOmega)
  max S/1(maxS) -> product/3, Scope2/1
  Г(z)/1 -> max S/4(gammaZ)
  z/1 -> max S/2(z)
  ||Ω||/1(normOmega) -> "||Ω|| >= Ω cap ? "/1
  Ω * √n/1 -> "||Ω|| >= Ω cap ? "/2, Ω / Ω cap/2
  "||Ω|| >= Ω cap ? "/1 -> Ψ/1(isGreater)
  Ψ/1(Psi) -> product/1
  Ω / Ω cap/1 -> product/2
  product/1 -> Unary Minus/1
  Unary Minus/1 -> Fc/1
  Clock/1 -> max S/5(t)
  mu/1 -> max S/6(mu)

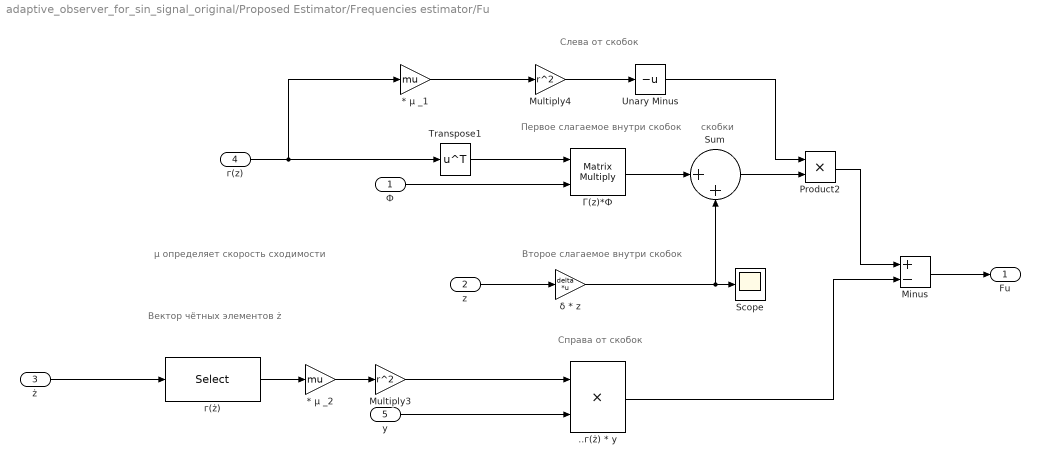
== system adaptive_observer_for_sin_signal_original/Proposed Estimator/Frequencies estimator/Fu ==
  note: Вектор чётных элементов ż
  note: μ определяет скорость сходимости
  note: скобки
  note: Первое слагаемое внутри скобок
  note: Второе слагаемое внутри скобок
  note: Слева от скобок
  note: Справа от скобок
  Ф : Inport
  z : Inport  Port=2
  ż : Inport  Port=3
  г(z) : Inport  Port=4
  y : Inport  Port=5
  * μ _1 : Gain  Gain=mu
  * μ _2 : Gain  Gain=mu
  ..г(ż) * y : Product
  Minus : Sum  Inputs=+-
  Multiply3 : Gain  Gain=r^2
  Multiply4 : Gain  Gain=r^2
  Product2 : Product
  Scope : Scope
  Sum : Sum  Inputs=|++
  Transpose1 : Math  Operator=transpose  SaturateOnIntegerOverflow=on
  Unary Minus : UnaryMinus
  δ * z : Gain  Gain=delta  Multiplication=Matrix(K*u)
  Г(z)*Ф : Product  Multiplication=Matrix(*)
  г(ż) : Selector  InputPortWidth=2*dimension+1  IndexOptions=Index vector (dialog)  Indices=2:2:2*dimension  OutputSizes=1
  Fu : Outport
  wires:
  ż/1 -> г(ż)/1
  г(z)/1 -> * μ _1/1, Transpose1/1
  * μ _2/1 -> Multiply3/1
  г(ż)/1 -> * μ _2/1
  Multiply3/1 -> ..г(ż) * y/1
  y/1 -> ..г(ż) * y/2
  Transpose1/1 -> Г(z)*Ф/1
  * μ _1/1 -> Multiply4/1
  Multiply4/1 -> Unary Minus/1
  z/1 -> δ * z/1
  Г(z)*Ф/1 -> Sum/1
  δ * z/1 -> Scope/1, Sum/2
  Unary Minus/1 -> Product2/1
  Sum/1 -> Product2/2
  Product2/1 -> Minus/1
  ..г(ż) * y/1 -> Minus/2
  Minus/1 -> Fu/1
  Ф/1 -> Г(z)*Ф/2

== system adaptive_observer_for_sin_signal_original/Proposed Estimator/Frequencies estimator/Ω ==
  note: Оценка частот в момент времени t
  θ : Inport
  y : Inport  Port=2
  г(z) : Inport  Port=3
  ..г(z)*y : Product
  Gain : Gain  Gain=r^2
  Sum : Sum  Inputs=|++
  μ : Gain  Gain=mu
  Ω : Outport
  wires:
  г(z)/1 -> Gain/1
  Gain/1 -> μ/1
  μ/1 -> ..г(z)*y/1
  y/1 -> ..г(z)*y/2
  ..г(z)*y/1 -> Sum/1
  θ/1 -> Sum/2
  Sum/1 -> Ω/1

== system adaptive_observer_for_sin_signal_original/Proposed Estimator/Frequencies estimator/θ' ==
  note: Образует основу θ'
  note: Удерживает Ω в области определения
  Fu : Inport
  Fc : Inport  Port=2
  Sum : Sum  Inputs=|++
  θ' : Outport
  wires:
  Fu/1 -> Sum/2
  Sum/1 -> θ'/1
  Fc/1 -> Sum/1

== system adaptive_observer_for_sin_signal_original/Proposed Estimator/z'/S(z) ==
  zPreDot : Inport
  z : Inport  Port=2
  Constant : Constant  Value=0
  Constant1 : Constant  Value=zMax * r^2
  Divide : Product  Inputs=*/
  MATLAB Function : MATLAB Function  TreatAsAtomicUnit=on
  Product : Product  Multiplication=Matrix(*)
  Product1 : Product  Multiplication=Matrix(*)
  Product2 : Product
  Relational Operator : RelationalOperator  OutDataTypeStr=boolean  RndMeth=Simplest
  Relational Operator1 : RelationalOperator  Operator=>  OutDataTypeStr=boolean  RndMeth=Simplest
  Transpose : Math  Operator=transpose  SaturateOnIntegerOverflow=on
  Transpose1 : Math  Operator=transpose  SaturateOnIntegerOverflow=on
  Z limiter : Constant  Value=zMax * r^2
  normalize : MATLAB Function  TreatAsAtomicUnit=on
  valType filter : MATLAB Function  TreatAsAtomicUnit=on
  S : Outport
  wires:
  Z limiter/1 -> Relational Operator/2
  normalize/1(normZ) -> Relational Operator/1
  Relational Operator/1 -> MATLAB Function/1(con1)
  z/1 -> Product1/1, Transpose1/1, Transpose/1, normalize/1(z)
  Transpose/1 -> Product/1
  zPreDot/1 -> Product/2
  Product/1 -> valType filter/1(multiplied)
  Constant/1 -> Relational Operator1/2
  Relational Operator1/1 -> MATLAB Function/2(con2)
  MATLAB Function/1(res) -> Product2/1
  Transpose1/1 -> Product1/2
  Product1/1 -> Product2/2
  Product2/1 -> Divide/1
  Constant1/1 -> Divide/2
  Divide/1 -> S/1
  valType filter/1(filtered) -> Relational Operator1/1

== system adaptive_observer_for_sin_signal_original/Proposed Estimator/z'/Subsystem ==
  bigGamma : Inport
  PHI : Inport  Port=2
  y : Inport  Port=3
  z : Inport  Port=4
  C : Constant  Value=C
  Const Matrix : Constant  Value=A
  L : Constant  Value=L
  Minus : Sum  Inputs=+-
  Product{,1..3} (4 alike) : Product  Multiplication=Matrix(*)
  Sum : Sum  Inputs=|+++
  Transpose : Math  Operator=transpose  SaturateOnIntegerOverflow=on
  Transpose1 : Math  Operator=transpose  SaturateOnIntegerOverflow=on
  Transpose2 : Math  Operator=transpose  SaturateOnIntegerOverflow=on
  zPreDot : Outport
  wires:
  z/1 -> Product2/2, Product/2
  Sum/1 -> zPreDot/1
  C/1 -> Transpose/1
  y/1 -> Minus/1
  Product/1 -> Minus/2
  L/1 -> Transpose1/1
  Minus/1 -> Product1/2
  Const Matrix/1 -> Product2/1
  bigGamma/1 -> Product3/1
  PHI/1 -> Product3/2
  Product2/1 -> Sum/1
  Product3/1 -> Sum/2
  Product1/1 -> Sum/3
  Transpose/1 -> Product/1
  Transpose2/1 -> Product1/1
  Transpose1/1 -> Transpose2/1

== system adaptive_observer_for_sin_signal_original/Proposed Estimator1/Frequencies estimator/Fc ==
  note: Определение максимального S
  note: Переключатель ограничителя Fc
  z : Inport
  Ω : Inport  Port=2
  Ф : Inport  Port=3
  Г(z) : Inport  Port=4
  Clock : Clock
  Scope2 : Scope
  Unary Minus : UnaryMinus
  max S : MATLAB Function  TreatAsAtomicUnit=on
  mu : Constant  Value=mu
  product : Product  Inputs=3
  ||Ω|| : MATLAB Function  TreatAsAtomicUnit=on
  "||Ω|| >= Ω cap ? " : RelationalOperator  OutDataTypeStr=boolean  RndMeth=Simplest
  Ψ : MATLAB Function  TreatAsAtomicUnit=on
  Ω * √n : Constant  Value=omegaLimiter
  Ω / Ω cap : Product  Inputs=*/
  Fc : Outport
  wires:
  Ф/1 -> max S/3(PHI)
  Ω/1 -> max S/1(bigOmega), Ω / Ω cap/1, ||Ω||/1(bigOmega)
  max S/1(maxS) -> product/3, Scope2/1
  Г(z)/1 -> max S/4(gammaZ)
  z/1 -> max S/2(z)
  ||Ω||/1(normOmega) -> "||Ω|| >= Ω cap ? "/1
  Ω * √n/1 -> "||Ω|| >= Ω cap ? "/2, Ω / Ω cap/2
  "||Ω|| >= Ω cap ? "/1 -> Ψ/1(isGreater)
  Ψ/1(Psi) -> product/1
  Ω / Ω cap/1 -> product/2
  product/1 -> Unary Minus/1
  Unary Minus/1 -> Fc/1
  Clock/1 -> max S/5(t)
  mu/1 -> max S/6(mu)

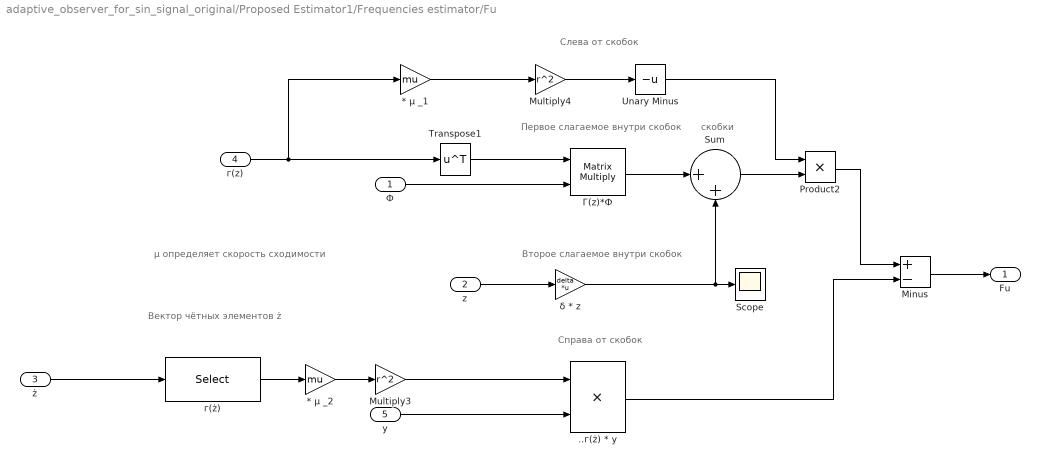
== system adaptive_observer_for_sin_signal_original/Proposed Estimator1/Frequencies estimator/Fu ==
  note: Вектор чётных элементов ż
  note: μ определяет скорость сходимости
  note: скобки
  note: Первое слагаемое внутри скобок
  note: Второе слагаемое внутри скобок
  note: Слева от скобок
  note: Справа от скобок
  Ф : Inport
  z : Inport  Port=2
  ż : Inport  Port=3
  г(z) : Inport  Port=4
  y : Inport  Port=5
  * μ _1 : Gain  Gain=mu
  * μ _2 : Gain  Gain=mu
  ..г(ż) * y : Product
  Minus : Sum  Inputs=+-
  Multiply3 : Gain  Gain=r^2
  Multiply4 : Gain  Gain=r^2
  Product2 : Product
  Scope : Scope
  Sum : Sum  Inputs=|++
  Transpose1 : Math  Operator=transpose  SaturateOnIntegerOverflow=on
  Unary Minus : UnaryMinus
  δ * z : Gain  Gain=delta  Multiplication=Matrix(K*u)
  Г(z)*Ф : Product  Multiplication=Matrix(*)
  г(ż) : Selector  InputPortWidth=2*dimension+1  IndexOptions=Index vector (dialog)  Indices=2:2:2*dimension  OutputSizes=1
  Fu : Outport
  wires:
  ż/1 -> г(ż)/1
  г(z)/1 -> * μ _1/1, Transpose1/1
  * μ _2/1 -> Multiply3/1
  г(ż)/1 -> * μ _2/1
  Multiply3/1 -> ..г(ż) * y/1
  y/1 -> ..г(ż) * y/2
  Transpose1/1 -> Г(z)*Ф/1
  * μ _1/1 -> Multiply4/1
  Multiply4/1 -> Unary Minus/1
  z/1 -> δ * z/1
  Г(z)*Ф/1 -> Sum/1
  δ * z/1 -> Scope/1, Sum/2
  Unary Minus/1 -> Product2/1
  Sum/1 -> Product2/2
  Product2/1 -> Minus/1
  ..г(ż) * y/1 -> Minus/2
  Minus/1 -> Fu/1
  Ф/1 -> Г(z)*Ф/2

== system adaptive_observer_for_sin_signal_original/Proposed Estimator1/Frequencies estimator/Ω ==
  note: Оценка частот в момент времени t
  θ : Inport
  y : Inport  Port=2
  г(z) : Inport  Port=3
  ..г(z)*y : Product
  Gain : Gain  Gain=r^2
  Sum : Sum  Inputs=|++
  μ : Gain  Gain=mu
  Ω : Outport
  wires:
  г(z)/1 -> Gain/1
  Gain/1 -> μ/1
  μ/1 -> ..г(z)*y/1
  y/1 -> ..г(z)*y/2
  ..г(z)*y/1 -> Sum/1
  θ/1 -> Sum/2
  Sum/1 -> Ω/1

== system adaptive_observer_for_sin_signal_original/Proposed Estimator1/Frequencies estimator/θ' ==
  note: Образует основу θ'
  note: Удерживает Ω в области определения
  Fu : Inport
  Fc : Inport  Port=2
  Sum : Sum  Inputs=|++
  θ' : Outport
  wires:
  Fu/1 -> Sum/2
  Sum/1 -> θ'/1
  Fc/1 -> Sum/1

== system adaptive_observer_for_sin_signal_original/Proposed Estimator1/z'/S(z) ==
  zPreDot : Inport
  z : Inport  Port=2
  Constant : Constant  Value=0
  Constant1 : Constant  Value=zMax * r^2
  Divide : Product  Inputs=*/
  MATLAB Function : MATLAB Function  TreatAsAtomicUnit=on
  Product : Product  Multiplication=Matrix(*)
  Product1 : Product  Multiplication=Matrix(*)
  Product2 : Product
  Relational Operator : RelationalOperator  OutDataTypeStr=boolean  RndMeth=Simplest
  Relational Operator1 : RelationalOperator  Operator=>  OutDataTypeStr=boolean  RndMeth=Simplest
  Transpose : Math  Operator=transpose  SaturateOnIntegerOverflow=on
  Transpose1 : Math  Operator=transpose  SaturateOnIntegerOverflow=on
  Z limiter : Constant  Value=zMax * r^2
  normalize : MATLAB Function  TreatAsAtomicUnit=on
  S : Outport
  wires:
  Z limiter/1 -> Relational Operator/2
  normalize/1(normZ) -> Relational Operator/1
  Relational Operator/1 -> MATLAB Function/1(con1)
  z/1 -> Product1/1, Transpose1/1, Transpose/1, normalize/1(z)
  Transpose/1 -> Product/1
  zPreDot/1 -> Product/2
  Constant/1 -> Relational Operator1/2
  Relational Operator1/1 -> MATLAB Function/2(con2)
  MATLAB Function/1(res) -> Product2/1
  Transpose1/1 -> Product1/2
  Product1/1 -> Product2/2
  Product2/1 -> Divide/1
  Constant1/1 -> Divide/2
  Divide/1 -> S/1
  Product/1 -> Relational Operator1/1

== system adaptive_observer_for_sin_signal_original/Proposed Estimator1/z'/Subsystem ==
  bigGamma : Inport
  PHI : Inport  Port=2
  y : Inport  Port=3
  z : Inport  Port=4
  C : Constant  Value=C
  Const Matrix : Constant  Value=A
  L : Constant  Value=L1
  Minus : Sum  Inputs=+-
  Product{,1..3} (4 alike) : Product  Multiplication=Matrix(*)
  Sum : Sum  Inputs=|+++
  Transpose : Math  Operator=transpose  SaturateOnIntegerOverflow=on
  Transpose1 : Math  Operator=transpose  SaturateOnIntegerOverflow=on
  Transpose2 : Math  Operator=transpose  SaturateOnIntegerOverflow=on
  zPreDot : Outport
  wires:
  z/1 -> Product2/2, Product/2
  Sum/1 -> zPreDot/1
  C/1 -> Transpose/1
  y/1 -> Minus/1
  Product/1 -> Minus/2
  L/1 -> Transpose1/1
  Minus/1 -> Product1/2
  Const Matrix/1 -> Product2/1
  bigGamma/1 -> Product3/1
  PHI/1 -> Product3/2
  Product2/1 -> Sum/1
  Product3/1 -> Sum/2
  Product1/1 -> Sum/3
  Transpose/1 -> Product/1
  Transpose2/1 -> Product1/1
  Transpose1/1 -> Transpose2/1

== matlab function adaptive_observer_for_sin_signal_original/Estimator mu=5/Frequencies estimator/Fc/max S1 ==
  settings: sampleTime=0.1
  data: bigOmega input size=[dimension 1]; z input size=[2*dimension+1 1]; r parameter size=1; delta parameter size=[1 2*dimension+1]; PHI input size=[dimension 1]; maxS output size=1; gammaZ input size=[dimension 1]; t input size=1; dimension parameter size=1; mu input size=1
function maxS = SCounter(bigOmega, z, r, delta, PHI, gammaZ, t, dimension,...
mu)

    tempSum = 0;

    z2 = z(2:2:end);

    frequency = zeros(dimension,1);
    parfor i = 1:dimension
        frequency(i) = sqrt(abs(bigOmega(i))); 
    end

    
    if(t > 60 && t < 140)
        disturbanceDot = 1;
    else 
        disturbanceDot = 0;
    end

    parfor i = 1:dimension
        tempSum = tempSum + frequency(i)^2 * z2(i) + disturbanceDot; %1 
    end

    gammaZ = gammaZ';


    maxS = norm(r^2 * mu * gammaZ * tempSum - r^2 * mu * gammaZ ... 
       * (gammaZ * PHI + delta * z));


    maxS = maxS*1.1;

end

== matlab function adaptive_observer_for_sin_signal_original/Estimator mu=2.5/Frequencies estimator/Fc/||Ω|| ==
  data: bigOmega input size=[dimension 1]; normOmega output size=1
function normOmega = norma(bigOmega)

normOmega = norm(bigOmega);

== matlab function adaptive_observer_for_sin_signal_original/Proposed Estimator/Frequencies estimator/Fc/max S ==
  settings: sampleTime=0.1
  data: bigOmega input size=[dimension 1]; z input size=[2*dimension+1 1]; r parameter size=1; delta parameter size=[1 2*dimension+1]; PHI input size=[dimension 1]; maxS output size=1; gammaZ input size=[dimension 1]; t input size=1; dimension parameter size=1; mu input size=1
function maxS = SCounter(bigOmega, z, r, delta, PHI, gammaZ, t, dimension,...
mu)

    tempSum = 0;

    z2 = z(2:2:end);

    frequency = zeros(dimension,1);
    parfor i = 1:dimension
        frequency(i) = sqrt(abs(bigOmega(i))); 
    end

    
    if(t > 60 && t < 140)
        disturbanceDot = 1;
    else 
        disturbanceDot = 0;
    end

    parfor i = 1:dimension
        tempSum = tempSum + frequency(i)^2 * z2(i) + disturbanceDot; %1 
    end

    gammaZ = gammaZ';


    maxS = norm(r^2 * mu * gammaZ * tempSum - r^2 * mu * gammaZ ... 
       * (gammaZ * PHI + delta * z));


    maxS = maxS*1.1;

end

== matlab function adaptive_observer_for_sin_signal_original/Estimator mu=2.5/Frequencies estimator/Fc/Ψ ==
  data: isGreater input; Psi output
function Psi = PSI(isGreater)

if isGreater
    Psi = 1;
else 
    Psi = 0;
end

== matlab function adaptive_observer_for_sin_signal_original/Estimator mu=2.5/Subsystem1/MATLAB Function ==
  data: zPrime input; z output; t input; initialZ parameter
function z = fcn(zPrime, t, initialZ)

if (t == 0)
    cont = [0, initialZ];
    
end

== matlab function adaptive_observer_for_sin_signal_original/MATLAB Function ==
  data: bigOmega input; omega_hat output
function omega_hat = fcn(bigOmega)

omega_hat = sqrt(abs(bigOmega));

== matlab function adaptive_observer_for_sin_signal_original/Estimator mu=2.5/z'/S(z)/MATLAB Function ==
  data: con1 input; res output; con2 input
function res = fcn(con1, con2)

if (con1 == true) && (con2 == true)
    res = 1;
else
    res = 0;
end

== matlab function adaptive_observer_for_sin_signal_original/Estimator mu=2.5/z'/S(z)/normalize ==
  data: z input size=[2*dimension+1 1]; normZ output size=1
function normZ = norma(z)

normZ = norm(z);

== matlab function adaptive_observer_for_sin_signal_original/Estimator mu=2.5/z'/S(z)/valType detector ==
  data: multiplied input; filtered output
function filtered = fcn(multiplied)

if class(multiplied) == 'double'
    filtered = multiplied;
elseif class(multiplied) == 'complex'
    filtered = abs(multiplied);
end

== matlab function adaptive_observer_for_sin_signal_original/Estimator mu=2.5/Г(z) ==
  settings: sampleTime=0.1
  data: z input size=[2*dimension+1 1]; bigGammaZ output size=[2*dimension+1 dimension]; dimension parameter size=1; bigGammaZ0 parameter size=[2*dimension+1 dimension]
function bigGammaZ = gms1(z, dimension, bigGammaZ0)

bigGammaZ = bigGammaZ0;
for i = 1:dimension
    bigGammaZ(2*i - 1,i) = z(2*i);
end

== matlab function adaptive_observer_for_sin_signal_original/MATLAB Function2 ==
  data: bigOmega input; omega_hat output
function omega_hat = fcn(bigOmega)

omega_hat = sqrt(abs(bigOmega));

== matlab function adaptive_observer_for_sin_signal_original/Estimator mu=10/Frequencies estimator/Fc/max S1 ==
  settings: sampleTime=0.1
  data: bigOmega input size=[dimension 1]; z input size=[2*dimension+1 1]; r parameter size=1; delta parameter size=[1 2*dimension+1]; PHI input size=[dimension 1]; maxS output size=1; gammaZ input size=[dimension 1]; t input size=1; dimension parameter size=1; mu input size=1
function maxS = SCounter(bigOmega, z, r, delta, PHI, gammaZ, t, dimension,...
mu)

    tempSum = 0;

    z2 = z(2:2:end);

    frequency = zeros(dimension,1);
    parfor i = 1:dimension
        frequency(i) = sqrt(abs(bigOmega(i))); 
    end

    
    if(t > 60 && t < 140)
        disturbanceDot = 1;
    else 
        disturbanceDot = 0;
    end

    parfor i = 1:dimension
        tempSum = tempSum + frequency(i)^2 * z2(i) + disturbanceDot; %1 
    end

    gammaZ = gammaZ';


    maxS = norm(r^2 * mu * gammaZ * tempSum - r^2 * mu * gammaZ ... 
       * (gammaZ * PHI + delta * z));


    maxS = maxS*1.1;

end

== matlab function adaptive_observer_for_sin_signal_original/Estimator mu=5/Frequencies estimator/Fc/||Ω|| ==
  data: bigOmega input size=[dimension 1]; normOmega output size=1
function normOmega = norma(bigOmega)

normOmega = norm(bigOmega);

== matlab function adaptive_observer_for_sin_signal_original/Estimator mu=5/Frequencies estimator/Fc/Ψ ==
  data: isGreater input; Psi output
function Psi = PSI(isGreater)

if isGreater
    Psi = 1;
else 
    Psi = 0;
end

== matlab function adaptive_observer_for_sin_signal_original/Estimator mu=5/Subsystem1/MATLAB Function ==
  data: zPrime input; z output; t input; initialZ parameter
function z = fcn(zPrime, t, initialZ)

if (t == 0)
    cont = [0, initialZ];
    
end

== matlab function adaptive_observer_for_sin_signal_original/Approximated Signal ==
  data: bigOmega input size=[dimension 1]; t input; r parameter size=1; dimension parameter size=1; z input size=[2*dimension+1 1]; sgn_value output
function sgn_value = sgnl_generated(bigOmega, t, r, dimension, z)

z3 = z(end);
z1 = z(1:2:end-1);
z2 = z(2:2:end);

bias = z3;



frequency = zeros(1, dimension);
amplitude = zeros(1, dimension);
phase = zeros (1, dimension);

sgn_value = bias;

for j=1:dimension
    frequency(j) = sqrt(abs(bigOmega(j)));

    amplitude(j) = sqrt(z1(j).^2 + ((frequency(j).^2/r^4).*z2(j).^2));

    phase(j) = angle((frequency(j)/r^2).*z2(j) + 1i*z1(j)) - mod(frequency(j)*t, 2*pi);
    
    phase(j) = mod(phase(j) + pi, 2*pi) - pi;

    sgn_value = (sgn_value + amplitude(j).*sin(frequency(j)*t + phase(j)));
end

== matlab function adaptive_observer_for_sin_signal_original/Estimator mu=5/z'/S(z)/MATLAB Function ==
  data: con1 input; res output; con2 input
function res = fcn(con1, con2)

if (con1 == true) && (con2 == true)
    res = 1;
else
    res = 0;
end

== matlab function adaptive_observer_for_sin_signal_original/Estimator mu=5/z'/S(z)/normalize ==
  data: z input size=[2*dimension+1 1]; normZ output size=1
function normZ = norma(z)

normZ = norm(z);

== matlab function adaptive_observer_for_sin_signal_original/Estimator mu=5/z'/S(z)/valType detector ==
  data: multiplied input; filtered output
function filtered = fcn(multiplied)

if class(multiplied) == 'double'
    filtered = multiplied;
elseif class(multiplied) == 'complex'
    filtered = abs(multiplied);
end

== matlab function adaptive_observer_for_sin_signal_original/Estimator mu=5/Г(z) ==
  settings: sampleTime=0.1
  data: z input size=[2*dimension+1 1]; bigGammaZ output size=[2*dimension+1 dimension]; dimension parameter size=1; bigGammaZ0 parameter size=[2*dimension+1 dimension]
function bigGammaZ = gms1(z, dimension, bigGammaZ0)

bigGammaZ = bigGammaZ0;
for i = 1:dimension
    bigGammaZ(2*i - 1,i) = z(2*i);
end

== matlab function adaptive_observer_for_sin_signal_original/MATLAB Function3 ==
  data: bigOmega input; omega_hat output
function omega_hat = fcn(bigOmega)

omega_hat = sqrt(abs(bigOmega));

== matlab function adaptive_observer_for_sin_signal_original/FT Ved/DREM/MATLAB Function1 ==
  data: psi input; PSI output; psi_d input; PHI output; phi input; phi_d input; Psi output; Phi output; con output
function [PSI, PHI, Psi, Phi, con] = fcn(psi, psi_d, phi, phi_d)

Psi = zeros(2,1); Phi = zeros(2);
Psi(1) = psi; Psi(2) = psi_d;
Phi(1, :) = phi; Phi(2, :) = phi_d;

AdjF = [Phi(2,2), -Phi(2,1); -Phi(1,2), Phi(1,1)]';
PSI = AdjF*Psi;
PHI = det(Phi);
con = cond(Phi);

== matlab function adaptive_observer_for_sin_signal_original/Estimator mu=10/Frequencies estimator/Fc/||Ω|| ==
  data: bigOmega input size=[dimension 1]; normOmega output size=1
function normOmega = norma(bigOmega)

normOmega = norm(bigOmega);

== matlab function adaptive_observer_for_sin_signal_original/Estimator mu=10/Frequencies estimator/Fc/Ψ ==
  data: isGreater input; Psi output
function Psi = PSI(isGreater)

if isGreater
    Psi = 1;
else 
    Psi = 0;
end

== matlab function adaptive_observer_for_sin_signal_original/Estimator mu=10/Subsystem1/MATLAB Function ==
  data: zPrime input; z output; t input; initialZ parameter
function z = fcn(zPrime, t, initialZ)

if (t == 0)
    cont = [0, initialZ];
    
end

== matlab function adaptive_observer_for_sin_signal_original/Estimator mu=10/z'/S(z)/MATLAB Function ==
  data: con1 input; res output; con2 input
function res = fcn(con1, con2)

if (con1 == true) && (con2 == true)
    res = 1;
else
    res = 0;
end

== matlab function adaptive_observer_for_sin_signal_original/Estimator mu=10/z'/S(z)/normalize ==
  data: z input size=[2*dimension+1 1]; normZ output size=1
function normZ = norma(z)

normZ = norm(z);

== matlab function adaptive_observer_for_sin_signal_original/Estimator mu=10/z'/S(z)/valType detector ==
  data: multiplied input; filtered output
function filtered = fcn(multiplied)

if class(multiplied) == 'double'
    filtered = multiplied;
elseif class(multiplied) == 'complex'
    filtered = abs(multiplied);
end
